simulink model "KalmanM"  (R2020a)
settings: Solver=ode4  StartTime=0.0  StopTime=20  FixedStep=0.1  RelTol=1e-3
values from neighbouring files (symbols this model uses):
  A = [0 1;     -k/m -b/m]    [Kalman.m]    (also in fcn.m; temtProp.m = [0 1;-g/l 0]; untitled2.m)
  A1 = [0 1;-k/m -c/m]    [temtProp.m]
  B = [0; 1/m]    [Kalman.m]    (also in fcn.m; temtProp.m = [0;1/(m*l^2)]; untitled2.m)
  B1 = [0;1/m]    [temtProp.m]
  C = [0 1]    [Kalman.m]    (also in fcn.m; temtProp.m = [1 0]; untitled2.m)
  c = 5    [temtProp.m]
  C1 = [1 0]    [temtProp.m]
  D = 0    [Kalman.m]    (also in temtProp.m; untitled2.m)
  D1 = 0    [temtProp.m]
  f = 10000    [temtProp.m]
  g = 10    [temtProp.m]
  k = 5    [Kalman.m]    (also in fcn.m; temtProp.m = 100; untitled2.m)
  l = 0.4    [temtProp.m]
  m = 10    [Kalman.m]    (also in fcn.m; temtProp.m; untitled2.m)
  Q = diag([0.1 0])    [Kalman.m]    (also in fcn.m = 0.001; temtProp.m = 0.001; untitled2.m = 0.001)
  R = 10    [Kalman.m]    (also in fcn.m = 0.0001; temtProp.m = 0.0001; untitled2.m = 1-e4)
  Ts = 0.1    [temtProp.m]    (also in untitled2.m = 0.01)
undefined symbols (not defined in the file or in its folder): Continuous, Time
libraries: simulink x4, ctrlSharedLib x2
settings Model: Creator=Aero-Asus  LastModifiedBy=Aero-Asus

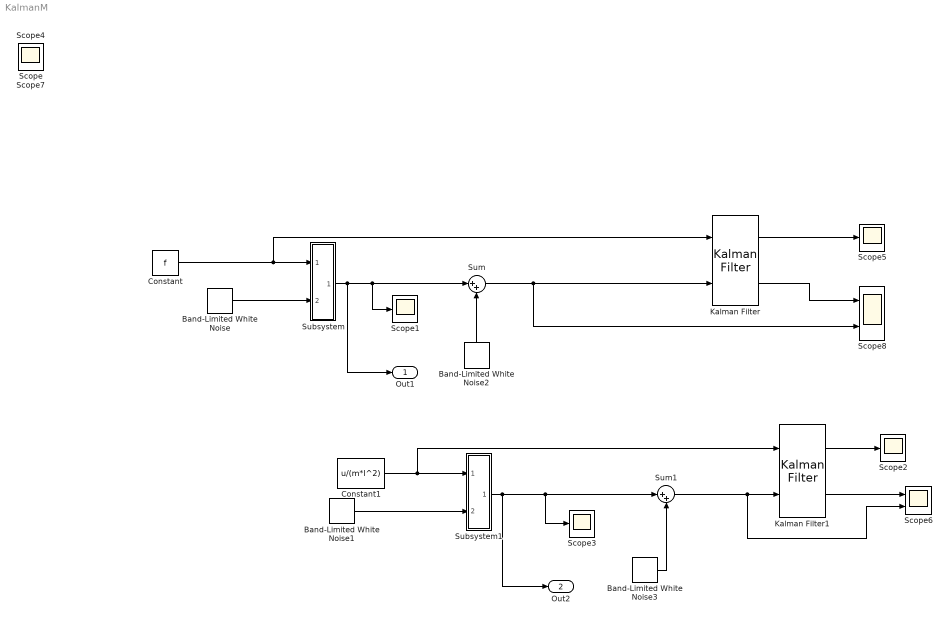
== system KalmanM ==
  Band-Limited White Noise : simulink/Sources/Band-Limited White Noise  Cov=Ts*R  Ts=Ts  seed=[23341]
  Band-Limited White Noise1 : simulink/Sources/Band-Limited White Noise  Cov=Ts*Q  Ts=Ts  seed=[23341]
  Band-Limited White Noise2 : simulink/Sources/Band-Limited White Noise  Cov=Ts*Q*1000  Ts=Ts  seed=[1000]
  Band-Limited White Noise3 : simulink/Sources/Band-Limited White Noise  Cov=Ts*Q  Ts=Ts  seed=[1000]
  Constant : Constant  Value=f
  Constant1 : Constant  Value=u/(m*l^2)
  Kalman Filter : ctrlSharedLib/Kalman Filter  TimeDomain=Continuous-Time  UseCurrentEstimator=on  ModelSource=Individual A, B, C, D matrices  ModelSourceVariable=ss(0.95,1,1,0,1)  A=A1  B=B1  C=C1  D=D1  NumberOfStates=1  NumberOfInputs=1  NumberOfOutputs=1  InitialEstimateSource=Dialog  X0=[0 0]  P0=10  UseK=off  UseGH=off  NumberOfProcessNoiseInputs=1  G=1  TimeInvariantG=on  H=0  TimeInvariantH=on  Q=diag([0 Q])  TimeInvariantQ=on  R=R  TimeInvariantR=on  N=0  TimeInvariantN=on  AddInputPort=on  AddEnablePort=off  OutputEstimatedY=on  OutputP=off  Ts=-1
  Kalman Filter1 : ctrlSharedLib/Kalman Filter  TimeDomain=Continuous-Time  UseCurrentEstimator=on  ModelSource=Individual A, B, C, D matrices  ModelSourceVariable=ss(0.95,1,1,0,1)  A=A  B=B  C=C  D=D  NumberOfStates=1  NumberOfInputs=1  NumberOfOutputs=1  InitialEstimateSource=Dialog  X0=[pi/18 0]  P0=10  UseK=off  UseGH=off  NumberOfProcessNoiseInputs=1  G=1  TimeInvariantG=on  H=0  TimeInvariantH=on  Q=diag([0 Q])  TimeInvariantQ=on  R=R  TimeInvariantR=on  N=0  TimeInvariantN=on  AddInputPort=on  AddEnablePort=off  OutputEstimatedY=on  OutputP=off  Ts=-1
  Scope{,1..5,7} (7 alike) : Scope
  Scope6 : Scope  NumInputPorts=2
  Scope8 : Scope  NumInputPorts=2
  Subsystem : Subsystem
  Subsystem1 : Subsystem
  Sum : Sum  Inputs=|++
  Sum1 : Sum  Inputs=|++
  Out1 : Outport
  Out2 : Outport  Port=2
  wires:
  Subsystem/1(Out1) -> Sum/1, Scope1/1, Out1/1
  Band-Limited White Noise/1 -> Subsystem/2(In2)
  Band-Limited White Noise1/1 -> Subsystem1/2(In2)
  Kalman Filter1/1 -> Scope2/1
  Subsystem1/1(Out1) -> Sum1/1, Scope3/1, Out2/1
  Constant1/1 -> Kalman Filter1/1, Subsystem1/1(In1)
  Sum/1 -> Kalman Filter/2, Scope8/2
  Band-Limited White Noise2/1 -> Sum/2
  Kalman Filter/1 -> Scope5/1
  Kalman Filter/2 -> Scope8/1
  Band-Limited White Noise3/1 -> Sum1/2
  Sum1/1 -> Scope6/2, Kalman Filter1/2
  Kalman Filter1/2 -> Scope6/1
  Constant/1 -> Subsystem/1(In1), Kalman Filter/1

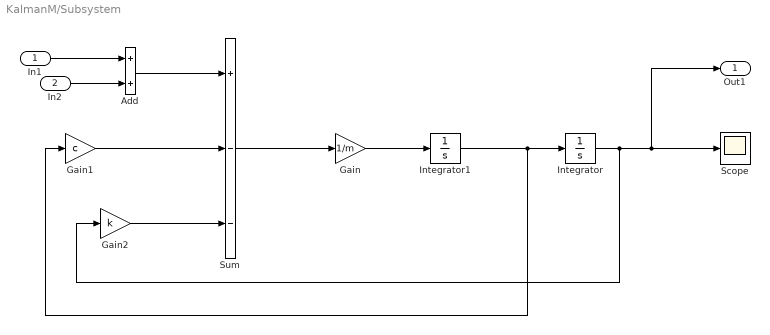
== system KalmanM/Subsystem ==
  In1 : Inport
  In2 : Inport  Port=2
  Add : Sum
  Gain : Gain  Gain=1/m
  Gain1 : Gain  Gain=c
  Gain2 : Gain  Gain=k
  Integrator : Integrator
  Integrator1 : Integrator
  Scope : Scope
  Sum : Sum  Inputs=+--
  Out1 : Outport
  wires:
  Integrator/1 -> Out1/1, Scope/1, Gain2/1
  Gain2/1 -> Sum/3
  Sum/1 -> Gain/1
  Integrator1/1 -> Gain1/1, Integrator/1
  Gain1/1 -> Sum/2
  Gain/1 -> Integrator1/1
  In1/1 -> Add/1
  In2/1 -> Add/2
  Add/1 -> Sum/1

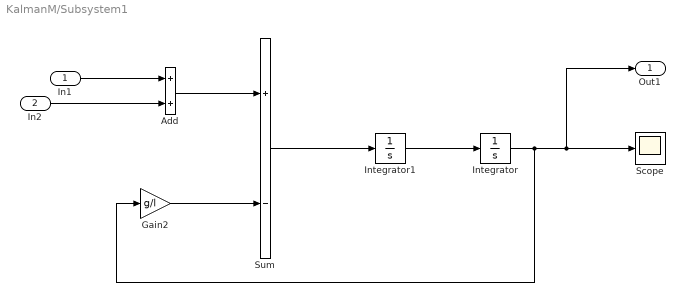
== system KalmanM/Subsystem1 ==
  In1 : Inport
  In2 : Inport  Port=2
  Add : Sum
  Gain2 : Gain  Gain=g/l
  Integrator : Integrator  InitialCondition=pi/18
  Integrator1 : Integrator
  Scope : Scope
  Sum : Sum  Inputs=+-
  Out1 : Outport
  wires:
  Add/1 -> Sum/1
  In2/1 -> Add/2
  In1/1 -> Add/1
  Sum/1 -> Integrator1/1
  Integrator1/1 -> Integrator/1
  Gain2/1 -> Sum/2
  Integrator/1 -> Gain2/1, Scope/1, Out1/1
